simulink model "FinalProject_simulink"  (R2019b)
settings: Solver=ode14x  StartTime=0.0  StopTime=10.0  FixedStep=0.001  RelTol=1e-3
values from neighbouring files (symbols this model uses):
  A = (A_given)*0.025400    [FinalProject.m]
  c1 = (c1_given)*175.127    (= 3502.54)    [FinalProject.m]
  E = (E_given)*0.025400    [FinalProject.m]
  k1 = (k1_given)*175.127    (= 21890.875)    [FinalProject.m]
  k2 = (k2_given)*175.127    (= 175127)    [FinalProject.m]
  m1 = (m1g)/9.81    (= 453.437308869)    [FinalProject.m]
  m1g = (m1g_given)*4.44822    (= 4448.22)    [FinalProject.m]
  m2 = (m2g)/9.81    (= 45.3437308869)    [FinalProject.m]
  m2g = (m2g_given)*4.44822    (= 444.822)    [FinalProject.m]
  P = (P_given)*0.025400    [FinalProject.m]
  v_slow = (v_slow_given)*0.44704    (= 6.7056)    [FinalProject.m]
settings Model: Creator=trevorhess  LastModifiedBy=trevorhess

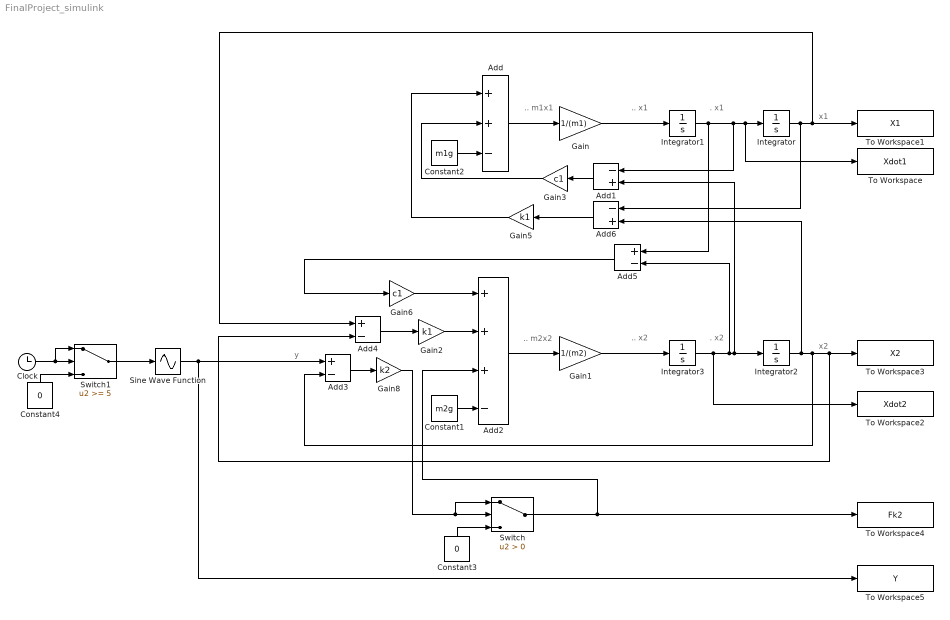
== system FinalProject_simulink ==
  note: ..
      | x1
  note: .
      | x1
  note: ..
      | m1x1
  note: x2
  note: .
      | x2
  note: x1
  note: y
  note: ..
      | m2x2
  note: ..
      | x2
  Add : Sum  Inputs=++-
  Add1 : Sum  Inputs=-+
  Add2 : Sum  Inputs=+++-
  Add3 : Sum  Inputs=+-
  Add4 : Sum  Inputs=+-
  Add5 : Sum  Inputs=+-
  Add6 : Sum  Inputs=-+
  Clock : Clock
  Constant1 : Constant  Value=m2g
  Constant2 : Constant  Value=m1g
  Constant3 : Constant  Value=0
  Constant4 : Constant  Value=0
  Gain : Gain  Gain=1/(m1)
  Gain1 : Gain  Gain=1/(m2)
  Gain2 : Gain  Gain=k1
  Gain3 : Gain  Gain=c1
  Gain5 : Gain  Gain=k1
  Gain6 : Gain  Gain=c1
  Gain8 : Gain  Gain=k2
  Integrator{,1..3} (4 alike) : Integrator
  Sine Wave Function : Sin  TimeSource=Use external signal  Amplitude=A  Bias=E  Frequency=((2*pi)/P)*v_slow  SampleTime=0
  Switch : Switch  Criteria=u2 > Threshold
  Switch1 : Switch  Threshold=5
  To Workspace : ToWorkspace  VariableName=Xdot1  SampleTime=-1
      settings: Save2DSignal=2-D array (concatenate along first dimension)
  To Workspace1 : ToWorkspace  VariableName=X1  SampleTime=-1
      settings: Save2DSignal=2-D array (concatenate along first dimension)
  To Workspace2 : ToWorkspace  VariableName=Xdot2  SampleTime=-1
      settings: Save2DSignal=2-D array (concatenate along first dimension)
  To Workspace3 : ToWorkspace  VariableName=X2  SampleTime=-1
      settings: Save2DSignal=2-D array (concatenate along first dimension)
  To Workspace4 : ToWorkspace  VariableName=Fk2  SampleTime=-1
      settings: Save2DSignal=2-D array (concatenate along first dimension)
  To Workspace5 : ToWorkspace  VariableName=Y  SampleTime=-1
      settings: Save2DSignal=2-D array (concatenate along first dimension)
  wires:
  Add4/1 -> Gain2/1
  Add1/1 -> Gain3/1
  Integrator3/1 -> Add5/2, Add1/2, Integrator2/1, To Workspace2/1
  Add5/1 -> Gain6/1
  Add2/1 -> Gain1/1
  Gain1/1 -> Integrator3/1
  Add3/1 -> Gain8/1
  Integrator2/1 -> Add6/2, Add3/2, Add4/2, To Workspace3/1
  Gain/1 -> Integrator1/1
  Gain2/1 -> Add2/2
  Constant2/1 -> Add/3
  Integrator/1 -> Add6/1, Add4/1, To Workspace1/1
  Constant1/1 -> Add2/4
  Add/1 -> Gain/1
  Gain6/1 -> Add2/1
  Integrator1/1 -> To Workspace/1, Integrator/1, Add1/1, Add5/1
  Gain8/1 -> Switch/2, Switch/1
  Constant3/1 -> Switch/3
  Switch/1 -> Add2/3, To Workspace4/1
  Add6/1 -> Gain5/1
  Gain5/1 -> Add/1
  Gain3/1 -> Add/2
  Constant4/1 -> Switch1/3
  Switch1/1 -> Sine Wave Function/1
  Sine Wave Function/1 -> To Workspace5/1, Add3/1
  Clock/1 -> Switch1/1, Switch1/2
